simulink model "hexAero"  (R2024a)
settings: Solver=VariableStepAuto  StartTime=0.0  StopTime=10.0  RelTol=1e-3
undefined symbols (not defined in the file): vehicleParams
libraries: aerolibasang x1
settings Model: Creator=jerem  LastModifiedBy=GTAR

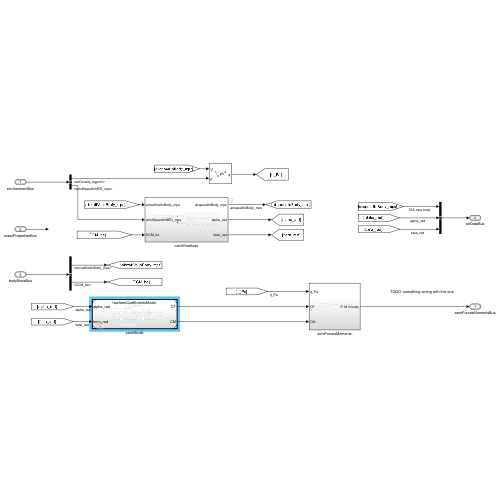
[thumbnail: Simulink's stored preview of the top-level diagram]
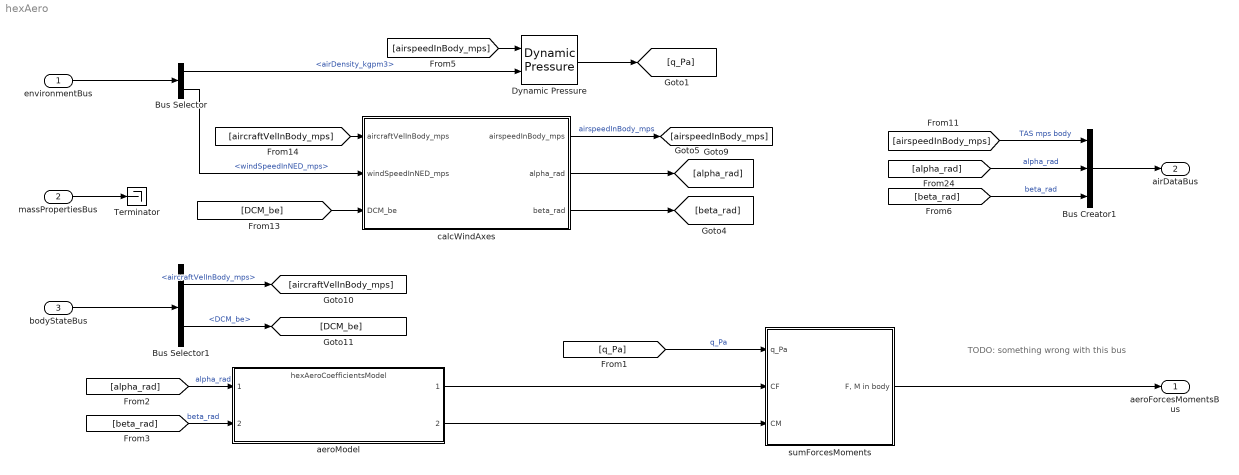
== system hexAero ==
  note: TODO: something wrong with this bus
  environmentBus : Inport  OutDataTypeStr=Bus: EnvironmentBus
  massPropertiesBus : Inport  Port=2  OutDataTypeStr=Bus: MassPropertiesBus
  bodyStateBus : Inport  Port=3  OutDataTypeStr=Bus: BodyStateBus
  Bus Creator1 : BusCreator  Inputs=3
  Bus Selector : BusSelector  OutputSignals=AirEnvironment.airDensity_kgpm3,AirEnvironment.windSpeedInNED_mps
  Bus Selector1 : BusSelector  OutputSignals=aircraftVelInBody_mps,DCM_be
  Dynamic Pressure : aerolibasang/Dynamic Pressure
  Terminator : Terminator
  aeroModel : ModelReference  ModelNameDialog=hexAeroCoefficientsModel  SimulationMode=Normal  ModelReferenceVersion=1.5
  calcWindAxes : Subsystem
  sumForcesMoments : Subsystem
  aeroForcesMomentsBus : Outport  OutDataTypeStr=Bus: ComponentForcesMomentsBus
  airDataBus : Outport  Port=2  OutDataTypeStr=Bus: AirData
  wires:
  Bus Creator1/1 -> airDataBus/1
  [alpha_rad] -> Bus Creator1/2  "alpha_rad"
  [airspeedInBody_mps] -> Bus Creator1/1  "TAS mps body"
  [beta_rad] -> Bus Creator1/3  "beta_rad"
  Bus Selector/2 -> calcWindAxes/2(windSpeedInNED_mps)  "<windSpeedInNED_mps>"
  Bus Selector/1 -> Dynamic Pressure/2  "<airDensity_kgpm3>"
  environmentBus/1 -> Bus Selector/1
  Bus Selector1/2 -> [DCM_be]  "<DCM_be>"
  Bus Selector1/1 -> [aircraftVelInBody_mps]  "<aircraftVelInBody_mps>"
  bodyStateBus/1 -> Bus Selector1/1
  Dynamic Pressure/1 -> [q_Pa]
  [airspeedInBody_mps] -> Dynamic Pressure/1
  calcWindAxes/2(alpha_rad) -> [alpha_rad]
  calcWindAxes/3(beta_rad) -> [beta_rad]
  [aircraftVelInBody_mps] -> calcWindAxes/1(aircraftVelInBody_mps)
  calcWindAxes/1(airspeedInBody_mps) -> [airspeedInBody_mps]  "airspeedInBody_mps"
  [q_Pa] -> sumForcesMoments/1(q_Pa)  "q_Pa"
  sumForcesMoments/1("F, M in body") -> aeroForcesMomentsBus/1
  [DCM_be] -> calcWindAxes/3(DCM_be)
  aeroModel/1 -> sumForcesMoments/2(CF)
  [alpha_rad] -> aeroModel/1  "alpha_rad"
  [beta_rad] -> aeroModel/2  "beta_rad"
  aeroModel/2 -> sumForcesMoments/3(CM)
  massPropertiesBus/1 -> Terminator/1

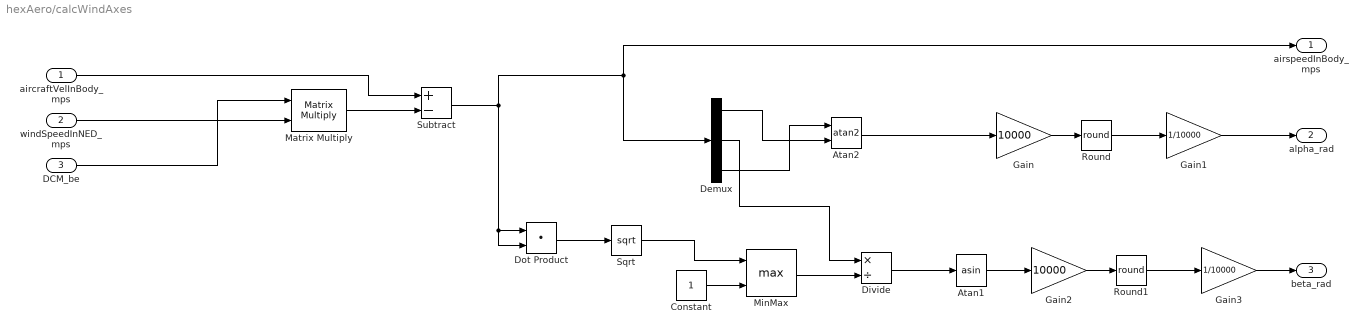
== system hexAero/calcWindAxes ==
  aircraftVelInBody_mps : Inport
  windSpeedInNED_mps : Inport  Port=2
  DCM_be : Inport  Port=3
  Atan1 : Trigonometry  Operator=asin
  Atan2 : Trigonometry  Operator=atan2
  Constant : Constant
  Demux : Demux  Outputs=3
  Divide : Product  Inputs=*/
  Dot Product : DotProduct  OutDataTypeStr=Inherit: Inherit via internal rule
  Gain : Gain  Gain=10000
  Gain1 : Gain  Gain=1/10000
  Gain2 : Gain  Gain=10000
  Gain3 : Gain  Gain=1/10000
  Matrix Multiply : Product  Multiplication=Matrix(*)
  MinMax : MinMax  Function=max  Inputs=2
  Round : Rounding  Operator=round
  Round1 : Rounding  Operator=round
  Sqrt : Sqrt
  Subtract : Sum  Inputs=+-
  airspeedInBody_mps : Outport
  alpha_rad : Outport  Port=2
  beta_rad : Outport  Port=3
  wires:
  DCM_be/1 -> Matrix Multiply/1
  windSpeedInNED_mps/1 -> Matrix Multiply/2
  Matrix Multiply/1 -> Subtract/2
  aircraftVelInBody_mps/1 -> Subtract/1
  Subtract/1 -> Dot Product/2, Dot Product/1, Demux/1, airspeedInBody_mps/1
  Dot Product/1 -> Sqrt/1
  Constant/1 -> MinMax/2
  Sqrt/1 -> MinMax/1
  MinMax/1 -> Divide/2
  Demux/2 -> Divide/1
  Divide/1 -> Atan1/1
  Demux/1 -> Atan2/2
  Demux/3 -> Atan2/1
  Atan2/1 -> Gain/1
  Gain/1 -> Round/1
  Round/1 -> Gain1/1
  Gain1/1 -> alpha_rad/1
  Round1/1 -> Gain3/1
  Gain2/1 -> Round1/1
  Atan1/1 -> Gain2/1
  Gain3/1 -> beta_rad/1

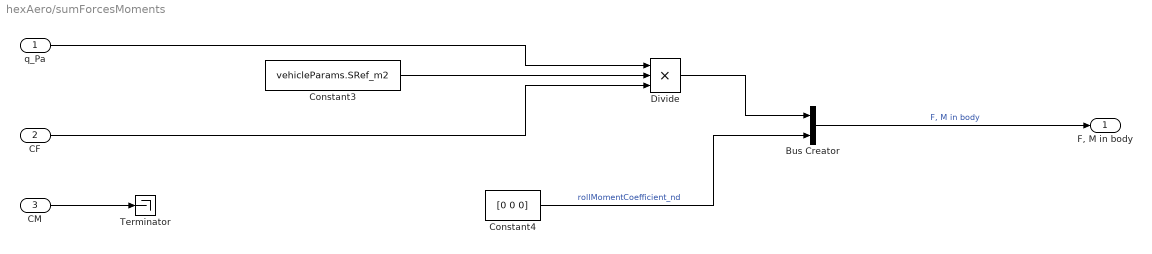
== system hexAero/sumForcesMoments ==
  q_Pa : Inport
  CF : Inport  Port=2
  CM : Inport  Port=3
  Bus Creator : BusCreator  Inputs=2
  Constant3 : Constant  Value=vehicleParams.SRef_m2
  Constant4 : Constant  Value=[0 0 0]
  Divide : Product  Inputs=***
  Terminator : Terminator
  "F, M in body" : Outport
  wires:
  Divide/1 -> Bus Creator/1
  q_Pa/1 -> Divide/1
  Constant3/1 -> Divide/2
  Bus Creator/1 -> "F, M in body"/1  "F, M in body"
  Constant4/1 -> Bus Creator/2  "rollMomentCoefficient_nd"
  CF/1 -> Divide/3
  CM/1 -> Terminator/1
